simulink model "RL_multi_controller_deploy"  (R2021a)
settings: configuration reference "Controller_Config_sim" (kept outside this file)
values from neighbouring files (symbols this model uses):
  rl_sample_rate = 4.0    [rl_data.sldd]
undefined symbols (not defined in the file or in its folder): ts_raspi
libraries: deeplib x2
settings Model: DataDictionary=rl_data.sldd  Creator=tshintai  LastModifiedBy=tshintai
settings ConfigSetRef: SourceName=Controller_Config_sim

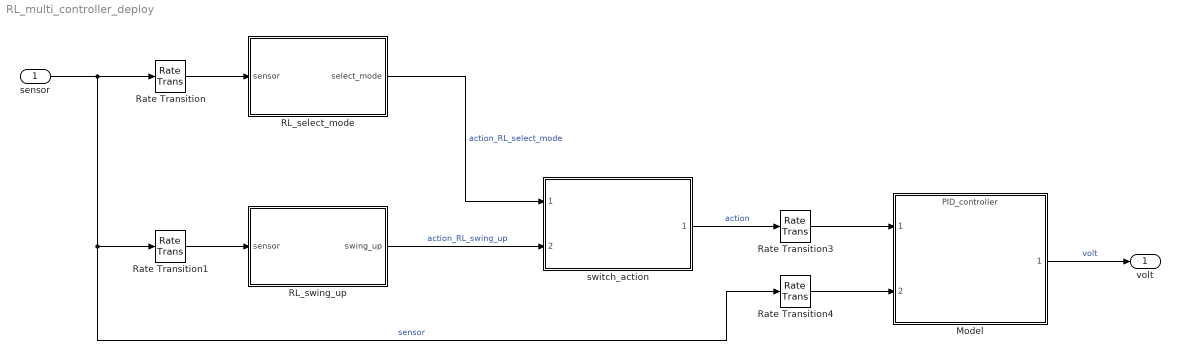
== system RL_multi_controller_deploy ==
  sensor : Inport  PortDimensions=4
  Model : ModelReference  ModelNameDialog=PID_controller.slx  SimulationMode=Normal  ModelReferenceVersion=1.63
  RL_select_mode : Subsystem
  RL_swing_up : Subsystem
  Rate Transition : RateTransition  OutPortSampleTime=ts_raspi*rl_sample_rate
  Rate Transition1 : RateTransition  OutPortSampleTime=ts_raspi*rl_sample_rate
  Rate Transition3 : RateTransition  OutPortSampleTime=ts_raspi
  Rate Transition4 : RateTransition  OutPortSampleTime=ts_raspi
  switch_action : Subsystem  ReferencedSubsystem=RL_multi_switch_action
  volt : Outport
  wires:
  Rate Transition/1 -> RL_select_mode/1(sensor)
  Rate Transition3/1 -> Model/1
  RL_select_mode/1(select_mode) -> switch_action/1  "action_RL_select_mode"
  Rate Transition4/1 -> Model/2
  sensor/1 -> Rate Transition1/1, Rate Transition4/1, Rate Transition/1  "sensor"
  switch_action/1 -> Rate Transition3/1  "action"
  Rate Transition1/1 -> RL_swing_up/1(sensor)
  RL_swing_up/1(swing_up) -> switch_action/2  "action_RL_swing_up"
  Model/1 -> volt/1  "volt"

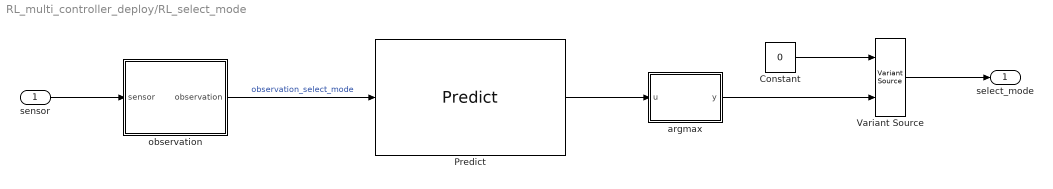
== system RL_multi_controller_deploy/RL_select_mode ==
  sensor : Inport
  Constant : Constant  Value=0
  Predict : deeplib/Predict  Network=Network from MAT-file  NetworkFunction=squeezenet  NetworkFilePath=policy_select.mat  MiniBatchSize=128  InputDataFormats={ '', '' }  Predictions=on  Activations={}  ForceInterpretedSim=off  EnableDLNetwork=on
      settings: SourceProductBaseCode=NN
  Variant Source : VariantSource
  argmax : MATLAB Function  TreatAsAtomicUnit=on
  "observation " : Subsystem  VariantControl=VARIANT_OBS_ARM_PEND
  select_mode : Outport
  wires:
  "observation "/1(observation) -> Predict/1  "observation_select_mode"
  sensor/1 -> "observation "/1(sensor)
  Variant Source/1 -> select_mode/1
  Constant/1 -> Variant Source/1
  Predict/1 -> argmax/1(u)
  argmax/1(y) -> Variant Source/2

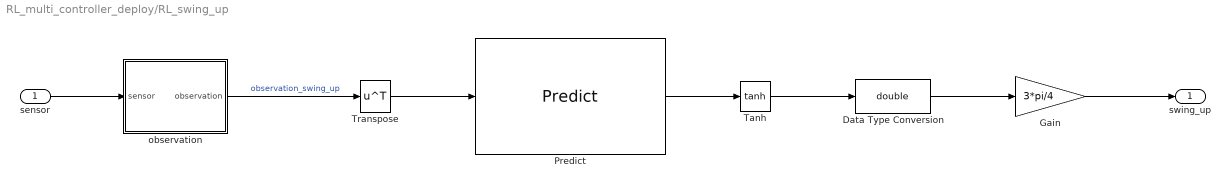
== system RL_multi_controller_deploy/RL_swing_up ==
  sensor : Inport
  Data Type Conversion : DataTypeConversion  OutDataTypeStr=double
  Gain : Gain  Gain=3*pi/4
  Predict : deeplib/Predict  Network=Network from MAT-file  NetworkFunction=squeezenet  NetworkFilePath=policy_swing.mat  MiniBatchSize=128  InputDataFormats={ '', '' }  Predictions=on  Activations={}  ForceInterpretedSim=off  EnableDLNetwork=on
      settings: SourceProductBaseCode=NN
  Tanh : Trigonometry  Operator=tanh
  Transpose : Math  Operator=transpose  SaturateOnIntegerOverflow=on
  "observation " : Subsystem  VariantControl=VARIANT_OBS_ARM_PEND
  swing_up : Outport
  wires:
  sensor/1 -> "observation "/1(sensor)
  "observation "/1(observation) -> Transpose/1  "observation_swing_up"
  Gain/1 -> swing_up/1
  Transpose/1 -> Predict/1
  Data Type Conversion/1 -> Gain/1
  Predict/1 -> Tanh/1
  Tanh/1 -> Data Type Conversion/1

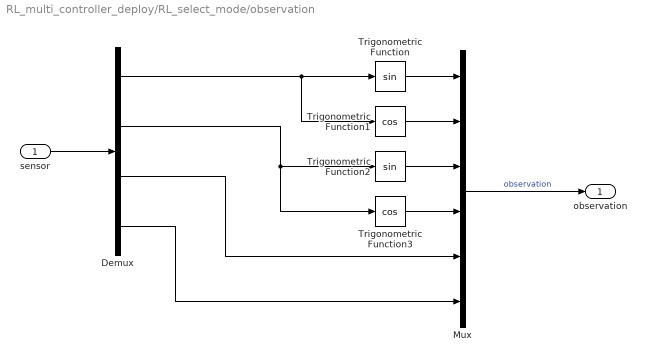
== system RL_multi_controller_deploy/RL_select_mode/observation  ==
  sensor : Inport
  Demux : Demux
  Mux : Mux  Inputs=6
  Trigonometric Function : Trigonometry
  Trigonometric Function1 : Trigonometry  Operator=cos
  Trigonometric Function2 : Trigonometry
  Trigonometric Function3 : Trigonometry  Operator=cos
  observation : Outport
  wires:
  Demux/3 -> Mux/5
  Demux/1 -> Trigonometric Function1/1, Trigonometric Function/1
  Trigonometric Function1/1 -> Mux/2
  Trigonometric Function/1 -> Mux/1
  Mux/1 -> observation/1  "observation"
  sensor/1 -> Demux/1
  Trigonometric Function2/1 -> Mux/3
  Trigonometric Function3/1 -> Mux/4
  Demux/2 -> Trigonometric Function3/1, Trigonometric Function2/1
  Demux/4 -> Mux/6

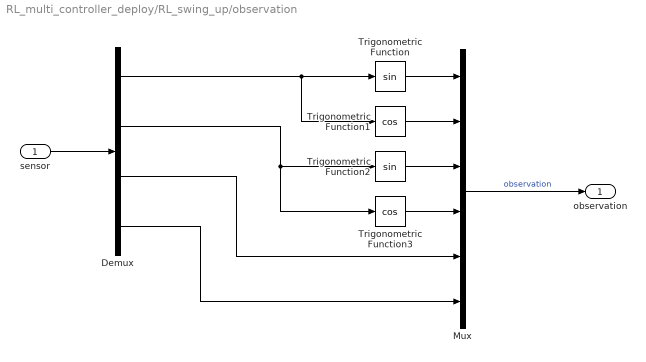
== system RL_multi_controller_deploy/RL_swing_up/observation  ==
  sensor : Inport
  Demux : Demux
  Mux : Mux  Inputs=6
  Trigonometric Function : Trigonometry
  Trigonometric Function1 : Trigonometry  Operator=cos
  Trigonometric Function2 : Trigonometry
  Trigonometric Function3 : Trigonometry  Operator=cos
  observation : Outport
  wires:
  Demux/4 -> Mux/6
  Demux/2 -> Trigonometric Function2/1, Trigonometric Function3/1
  Trigonometric Function3/1 -> Mux/4
  Trigonometric Function2/1 -> Mux/3
  sensor/1 -> Demux/1
  Mux/1 -> observation/1  "observation"
  Trigonometric Function/1 -> Mux/1
  Trigonometric Function1/1 -> Mux/2
  Demux/1 -> Trigonometric Function/1, Trigonometric Function1/1
  Demux/3 -> Mux/5

== matlab function RL_multi_controller_deploy/RL_select_mode/argmax ==
  data: u input; y output
function y = argmax(u)

[~, y] = max(u);
y = y - 1;

end
